simulink model "exampleStorage_type1_pipe_stratified"  (Simulink 7.6)
settings: Solver=ode45  StartTime=0.0  StopTime=3*3600-2  RelTol=1e-3
libraries: carnot x15, simulink x4
settings Model: Creator=drhf  LastModifiedBy=drhf
settings CodeAppCC: CustomSymbolStrType=$N$R$M_T

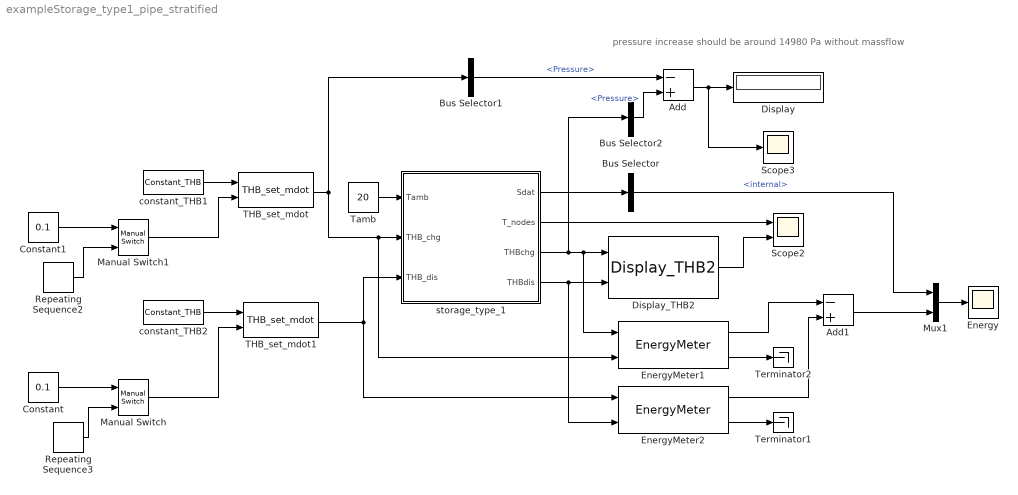
== system exampleStorage_type1_pipe_stratified ==
  note: pressure increase should be around 14980 Pa without massflow
  Add : Sum  Inputs=-+
  Add1 : Sum  Inputs=-+
  Bus Selector : BusSelector  OutputSignals=energy.internal
  Bus Selector1 : BusSelector  OutputSignals=Pressure
  Bus Selector2 : BusSelector  OutputSignals=Pressure
  Constant : Constant  Value=0.1
  Constant1 : Constant  Value=0.1
  Display : Display
  Display_THB2 : carnot/Outputs/Display_THB2  SystemSampleTime=-1  t=off  m=on  p=off  id=off  mix=off  d=off
  Energy : Scope
  EnergyMeter1 : carnot/Control/EnergyMeter  SystemSampleTime=-1
  EnergyMeter2 : carnot/Control/EnergyMeter  SystemSampleTime=-1
  Manual Switch : simulink/Signal Routing/Manual Switch  SystemSampleTime=-1  sw=0  action=0  varsize=off
  Manual Switch1 : simulink/Signal Routing/Manual Switch  SystemSampleTime=-1  sw=0  action=0  varsize=off
  Mux1 : Mux  Inputs=2
  Repeating Sequence2 : simulink/Sources/Repeating Sequence  SystemSampleTime=-1  rep_seq_t=[0 1 1 2 2 2.9 2.9 3.1]*3600  rep_seq_y=[0.12 0.12 0.15 0.15 0.1 0.1 0 0]
  Repeating Sequence3 : simulink/Sources/Repeating Sequence  SystemSampleTime=-1  rep_seq_t=[0 1 1 2 2 3]*3600  rep_seq_y=[0.12 0.12 0.1 0.1 0.15 0.15]
  Scope2 : Scope  NumInputPorts=2
      settings: YMin=-5~-5  YMax=5~5  SaveName=ScopeData3
  Scope3 : Scope
  THB_set_mdot : carnot/Source/Simple/THB_set_mdot  SystemSampleTime=-1
  THB_set_mdot1 : carnot/Source/Simple/THB_set_mdot  SystemSampleTime=-1
  Tamb : Constant  Value=20
  Terminator1 : Terminator
  Terminator2 : Terminator
  constant_THB1 : carnot/Source/Simple/Constant_THB  SystemSampleTime=-1  t=55  mdot=0*100/3600  p=1e5  mID=Full Pressure Drop with Static Height  fluid=water  mix=0  dia=0.02  hgt=0
  constant_THB2 : carnot/Source/Simple/Constant_THB  SystemSampleTime=-1  t=10  mdot=100/3600  p=1e5  mID=Full Pressure Drop with Static Height  fluid=water  mix=0  dia=0.02  hgt=0
  storage_type_1 : Subsystem  mask(Multiport Storage){uloss=0, ubot=0, utop=0, cond=1, tini=[20:5:65], volume=0.3, dia=0.5, pos=standing cylinder, nconnect=2, nodes=10, mpoints=10}
      mask prompts: uloss "Heat loss coefficient cylinder wall in W/(m²K)"; ubot "Heat loss coefficient bottom in W/(m²K)"; utop "Heat loss coefficient top cover in W/(m²K)"; cond "Effective vertical conductivity in W/(m*K)"; tini "Initial temperature (vector or scalar) in °C"; volume "Volume in m³"; dia "Diameter in m"; pos "Position"; nconnect "Number of connections"; nodes "Number of nodes"; mpoints "Number of measurement points"
      mask help:
      | The volmue of the cylindrical storage is divided in a number "nodes" of horizontal slices (1xN-node model). For each node the energy balance equation is solved.
      | Look under mask to set the ports types and properties.
      mask init:
      | standing = pos-1;
      | 
      | if standing
      |     dh = volume/(0.25*dia^2*pi*nodes);
      | else
      |     dh = dia/nodes;
      | end
      | 
      | % height = 0.5*dh : dh : dh*nodes;
      | height = dh*nodes;
      | 
      | mpoints = max(mpoints,1);
      | mpts = round(nodes/mpoints/2:nodes/mpoints:nodes);
      mask Help: eval('man(''storage_multiport'')')
      mask StyleString: edit,edit,edit,edit,edit,edit,edit,popup(lying cylinder|standing cylinder),edit,edit,edit
      mask TabNameString: Thermal,Thermal,Thermal,Thermal,Thermal,Geometry,Geometry,Geometry,Geometry,Calculation,Calculation
      mask Display: plot(10,10,90,100,[40,40,45,55,60,60,55,45,40],[84,36,30,30,36,84,90,90,84],[40,35],[77,77],[64,60],[77,77],[40,35],[42,42],[64,60],[42,42])
  wires:
  Bus Selector/1 -> Mux1/1  "<internal>"
  Tamb/1 -> storage_type_1/1(Tamb)
  THB_set_mdot/1 -> Bus Selector1/1, EnergyMeter1/2, storage_type_1/2(THB_chg)
  THB_set_mdot1/1 -> EnergyMeter2/1, storage_type_1/3(THB_dis)
  storage_type_1/1(Sdat) -> Bus Selector/1
  storage_type_1/2(T_nodes) -> Scope2/1
  storage_type_1/3(THBchg) -> Bus Selector2/1, Display_THB2/1, EnergyMeter1/1
  storage_type_1/4(THBdis) -> Display_THB2/2, EnergyMeter2/2
  Display_THB2/1 -> Scope2/2
  Mux1/1 -> Energy/1
  EnergyMeter2/2 -> Terminator1/1
  constant_THB1/1 -> THB_set_mdot/1
  constant_THB2/1 -> THB_set_mdot1/1
  Manual Switch1/1 -> THB_set_mdot/2
  Manual Switch/1 -> THB_set_mdot1/2
  Add/1 -> Display/1, Scope3/1
  Bus Selector1/1 -> Add/1  "<Pressure>"
  Bus Selector2/1 -> Add/2  "<Pressure>"
  Constant/1 -> Manual Switch/1
  Repeating Sequence3/1 -> Manual Switch/2
  Constant1/1 -> Manual Switch1/1
  Repeating Sequence2/1 -> Manual Switch1/2
  EnergyMeter1/2 -> Terminator2/1
  Add1/1 -> Mux1/2
  EnergyMeter2/1 -> Add1/2
  EnergyMeter1/1 -> Add1/1

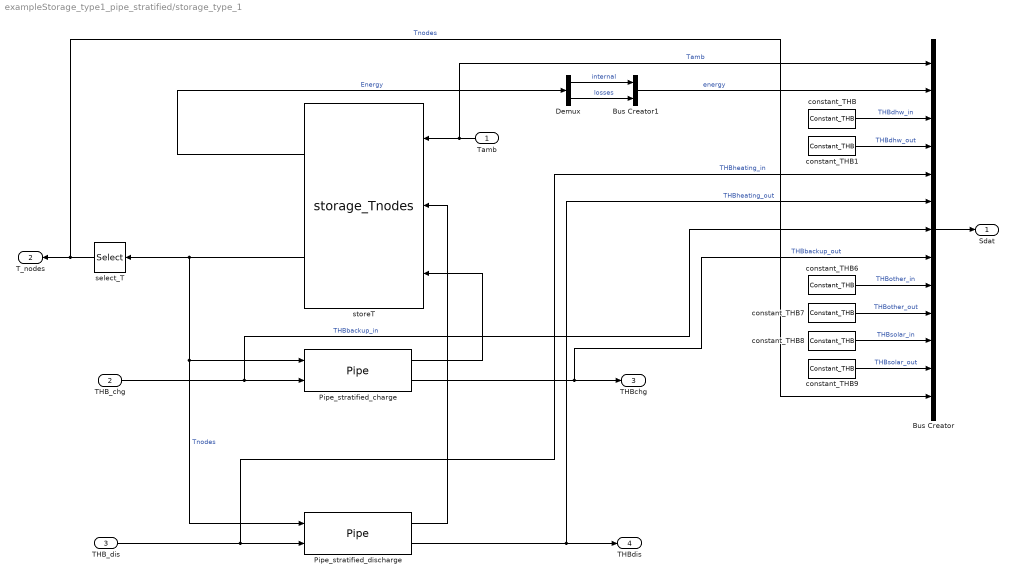
== system exampleStorage_type1_pipe_stratified/storage_type_1 ==
  Tamb : Inport
  THB_chg : Inport  Port=2
  THB_dis : Inport  Port=3
  Bus Creator : BusCreator  Inputs=13
  Bus Creator1 : BusCreator  Inputs=2
  Demux : Demux  Outputs=2
  Pipe_stratified_charge : carnot/Storage/Thermal/Storage_Ports/Pipe  SystemSampleTime=-1  h_in=1  h_out=0.2  dplin=0  dpqua=0  nodes=nodes  hgt=height  dia=dia
  Pipe_stratified_discharge : carnot/Storage/Thermal/Storage_Ports/Pipe  SystemSampleTime=-1  h_in=0  h_out=1  dplin=0  dpqua=0  nodes=nodes  hgt=height  dia=dia
  constant_THB{,1,6..9} (6 alike) : carnot/Source/Simple/Constant_THB  SystemSampleTime=-1  t=20  mdot=0  p=1e5  mID=No Pressure Drop  fluid=water  mix=0  dia=0.02  hgt=0
  select_T : Selector  InputPortWidth=nodes  IndexOptions=Index vector (dialog)  Indices=mpts  OutputSizes=1
  storeT : S-Function  FunctionName=storage_Tnodes  Parameters=dia, volume, standing, uloss , ubot, utop, cond, tini, nodes, nconnect  EnableBusSupport=off
  Sdat : Outport
  T_nodes : Outport  Port=2
  THBchg : Outport  Port=3
  THBdis : Outport  Port=4
  wires:
  Bus Creator1/1 -> Bus Creator/2  "energy"
  Demux/2 -> Bus Creator1/2  "losses"
  Demux/1 -> Bus Creator1/1  "internal"
  Pipe_stratified_charge/1 -> storeT/3
  Pipe_stratified_charge/2 -> Bus Creator/8, THBchg/1  "THBbackup_out"
  THB_chg/1 -> Bus Creator/7, Pipe_stratified_charge/2  "THBbackup_in"
  constant_THB6/1 -> Bus Creator/9  "THBother_in"
  constant_THB7/1 -> Bus Creator/10  "THBother_out"
  constant_THB8/1 -> Bus Creator/11  "THBsolar_in"
  constant_THB9/1 -> Bus Creator/12  "THBsolar_out"
  Bus Creator/1 -> Sdat/1
  constant_THB/1 -> Bus Creator/3  "THBdhw_in"
  constant_THB1/1 -> Bus Creator/4  "THBdhw_out"
  storeT/2 -> Pipe_stratified_discharge/1, Pipe_stratified_charge/1, select_T/1  "Tnodes"
  storeT/1 -> Demux/1  "Energy"
  select_T/1 -> Bus Creator/13, T_nodes/1  "Tnodes"
  Pipe_stratified_discharge/1 -> storeT/2
  Pipe_stratified_discharge/2 -> Bus Creator/6, THBdis/1  "THBheating_out"
  THB_dis/1 -> Bus Creator/5, Pipe_stratified_discharge/2  "THBheating_in"
  Tamb/1 -> Bus Creator/1, storeT/1  "Tamb"
